simulink model "SpeedGoat_GridModel"  (R2024a)
settings: Solver=FixedStepDiscrete  StartTime=0.0  StopTime=inf  RelTol=1e-3
StopFcn:
  | Root = pwd; PathTestResult = fullfile(Root, 'TestCases', 'TestResults'); ModelParam = struct(); if exist('Sim', 'var'), ModelParam.Sim = Sim; end; if exist('Hil', 'var'), ModelParam.Hil = Hil; end; if exist('out', 'var'),     saveTestResults(out, 'Speedgoat', 'Meas', PathTestResult, 1, ModelParam); else,     disp('Warning: Simulation output "out" not found in workspace after stop.'); end
values from neighbouring files (symbols this model uses):
  Hil = 100.0    [ModelDD.sldd]
  Sim : value not decoded    [ModelDD.sldd]
undefined symbols (not defined in the file or in its folder): DiscIntNeverNeededParam, Ended, IO324, IO3xx, pull, Single, up
libraries: speedgoatlib_fpga_pwm x5, speedgoatlib_fpga_analog_io x5, speedgoatlib_fpga_dio x3, simulink x3, speedgoatlib_fpga_inta x1, speedgoatlib_interrupt x1, speedgoatlib_fpga_quadrature x1, speedgoatlib_fpga_spi x1, dspswit3 x1, slrealtimeloglib x1, slrealtimetgmanagement x1, simulink_extras x1
settings Model: SimulationMode=external  ExtModeEnableFloating=off  Creator=simon.beck  LastModifiedBy=The Professionals
settings SolverCC: ConcurrentTasks=on  PositivePriorityOrder=on
settings DataIOCC: LimitDataPoints=on  SaveFormat=StructureWithTime  SaveOutput=off  DSMLogging=off  StreamToWks=off  SaveTime=off
settings OptimizationCC: BlockReduction=off  OptimizeBlockIOStorage=off  BufferReuse=off  ReuseModelBlockBuffer=off
settings DebuggingCC: UnderspecifiedInitializationDetection=Classic  MergeDetectMultiDrivingBlocksExec=none  TasksWithSamePriorityMsg=none  ParameterDowncastMsg=warning  ParameterOverflowMsg=warning  FcnCallInpInsideContextMsg=warning  FrameProcessingCompatibilityMsg=warning  NonCurrentReleaseOperatingPointMsg=warning  SFUnexpectedBacktrackingDiag=warning  SFOutputUsedAsStateInMooreChartDiag=warning
settings HardwareCC: ProdBitPerLong=64  ProdLongLongMode=on  ProdHWDeviceType=Intel->x86-64 (Linux 64)
settings ModelReferenceCC: EnableRefExpFcnMdlSchedulingChecks=on  PropagateSignalLabelsOutOfModel=off
settings RTWCC: Description=Speedgoat Real-Time Target Machine  SystemTargetFile=speedgoat.tlc  TemplateMakefile=slrealtime_default_tmf  PostCodeGenCommand=sg.model.build.makeCfg(bdroot, buildInfo);  Toolchain=Simulink Real-Time Toolchain  BuildConfiguration=Faster Runs  CodeExecutionProfiling=on  TargetLang=C++  GPUComputeCapability=3.5
settings SimulinkRealTimeTargetCC: InstructionSetFMA=off  LogToMDFFile=off

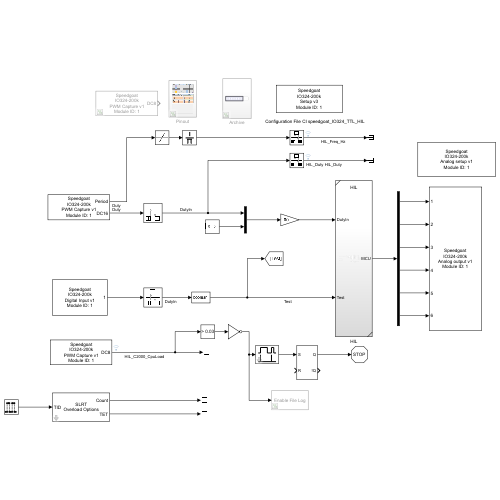
[thumbnail: Simulink's stored preview of the top-level diagram]
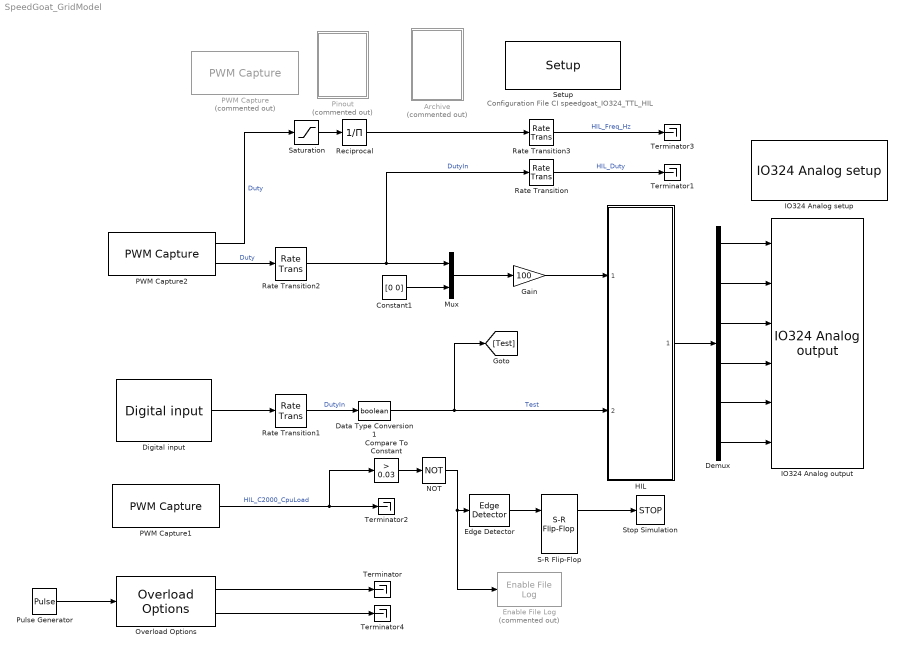
== system SpeedGoat_GridModel ==
  note: Configuration File CI speedgoat_IO324_TTL_HIL
  Archive : Subsystem  Commented=on
  Compare To Constant : simulink/Logic and Bit Operations/Compare To Constant  relop=>  const=0.03  OutDataTypeStr=boolean
  Constant1 : Constant  Value=[0 0]
  Data Type Conversion1 : DataTypeConversion  OutDataTypeStr=boolean  SaturateOnIntegerOverflow=off  RndMeth=Floor
  Demux : Demux  Outputs=6
  Digital input : speedgoatlib_fpga_dio/Digital input  id=1  chan=[1]  ts=1/Hil.PWM_Freq  vectorizeOutput=off
      settings: SourceProductName=Digital
  Edge Detector : dspswit3/Edge Detector  InputProcessing=Columns as channels (frame based)
  Enable File Log : slrealtimeloglib/Enable File Log  Commented=on
  Gain : Gain  Gain=100
  HIL : Subsystem  VariantControl="Sim.PlantOrMeas == \"HIL1\""  ReferencedSubsystem=HIL
  IO324 Analog output : speedgoatlib_fpga_analog_io/IO324/IO324 Analog output  id=1  parSampleTime=Sim.ContSampleTime  parPciSlot=-1  parAoChannels=[1 2 3 4 5 6]  parAoVoltageRange=[2 2 2 2 2 2]  parDacOverRange=[0 0 0 0 0 0 0 0]  parAoInitValues=[0 0 0 0 0 0]  parAoReset=[1 1 1 1 1 1]  parDacSyncOut=1  parAoEnableFrame=0  parDacActiveDmaDevices=[1 1 1 1]  parDacDmaLatency=2  parAoFrameSize=100
      settings: SourceProductName=Analog IO
  IO324 Analog setup : speedgoatlib_fpga_analog_io/IO324/IO324 Analog setup  id=1  parEnableCodeModule1=off  parEnableCodeModule2=off  parEnableCodeModule3=off  parEnableCodeModule4=off  parEnableCodeModule5=off  parEnableCodeModule6=off  parEnableCodeModule7=off  parEnableCodeModule8=off  parAdcEnableIndividualTrigger=off  parAdcTriggerMode1=Model Step  parAdcSampleRate1=100e3  parAdcDioTriggerChannel1=1  parAdcInternalTrigger1=<empty>  parAdcOversampling1=None  parAdcTriggerMode2=Model Step  parAdcSampleRate2=100e3  parAdcDioTriggerChannel2=1  parAdcInternalTrigger2=<empty>  parAdcOversampling2=None  parAdcTriggerMode3=Model Step  parAdcSampleRate3=100e3  parAdcDioTriggerChannel3=1  parAdcInternalTrigger3=<empty>  parAdcOversampling3=None  parAdcTriggerMode4=Model Step  parAdcSampleRate4=100e3  parAdcDioTriggerChannel4=1  parAdcInternalTrigger4=<empty>  parAdcOversampling4=None  parAdcReadPrevValueIndividualTrigger=on  parAdcEnableFrame=off  parAdcTriggerMode=Model Step  parAdcReadPrevValue=off  parAdcSampleRate=100e3  parAdcDioTriggerChannel=1  parAdcInternalTrigger=<empty>  parAdcOversampling=None  parAdcTriggerResolution=1e-08  parAdcSampleRateFrame=1000  parAdcFrameSize=100  parAdcSampleTime=-1  parDacTriggerMode=Model Step  parDacInternalTrigger=<empty>  parDacDioTriggerChannel=0  parDacEnableFrame=off  parDacFifoThreshold=100  parDacTriggerResolution=1e-08  parDacSampleRate=1000  parDacFrameSize=100  parDacSampleTime=-1  parAdcCoupling1=Differential  parAdcChannel1=on  parAdcChannel2=off  parAdcChannel3=on  parAdcChannel4=off  parAdcChannel5=off  parAdcChannel6=off  parAdcChannel7=off  parAdcChannel8=off  parAdcRangeAll1=+-10.24 V  parVoltageRangePerChannelEn1=off  parAdcRange1=+-10.24 V  parAdcRange5=+-10.24 V  parAdcRange2=+-10.24 V  parAdcRange6=+-10.24 V  parAdcRange3=+-10.24 V  parAdcRange7=+-10.24 V  parAdcRange4=+-10.24 V  parAdcRange8=+-10.24 V  parAdcCoupling2=Differential  parAdcChannel9=on  parAdcChannel10=off  parAdcChannel11=on  parAdcChannel12=off  parAdcChannel13=off  parAdcChannel14=off  parAdcChannel15=off  parAdcChannel16=off  parAdcRangeAll2=+-10.24 V  parVoltageRangePerChannelEn2=off  parAdcRange9=+-10.24 V  parAdcRange13=+-10.24 V  parAdcRange10=+-10.24 V  parAdcRange14=+-10.24 V  parAdcRange11=+-10.24 V  parAdcRange15=+-10.24 V  parAdcRange12=+-10.24 V  parAdcRange16=+-10.24 V  parAdcCoupling3=Single-Ended  parAdcChannel17=on  parAdcChannel18=on  parAdcChannel19=off  parAdcChannel20=off  parAdcChannel21=off  parAdcChannel22=off  parAdcChannel23=off  parAdcChannel24=off  parAdcRangeAll3=+-10.24 V  parVoltageRangePerChannelEn3=off  parAdcRange17=+-10.24 V  parAdcRange21=+-10.24 V  parAdcRange18=+-10.24 V  parAdcRange22=+-10.24 V  parAdcRange19=+-10.24 V  parAdcRange23=+-10.24 V  parAdcRange20=+-10.24 V  parAdcRange24=+-10.24 V  parAdcCoupling4=Single-Ended  parAdcChannel25=on  parAdcChannel26=on  parAdcChannel27=off  parAdcChannel28=off  parAdcChannel29=off  parAdcChannel30=off  parAdcChannel31=off  parAdcChannel32=off  parAdcRangeAll4=+-10.24 V  parVoltageRangePerChannelEn4=off  parAdcRange25=+-10.24 V  parAdcRange29=+-10.24 V  parAdcRange26=+-10.24 V  parAdcRange30=+-10.24 V  parAdcRange27=+-10.24 V  parAdcRange31=+-10.24 V  parAdcRange28=+-10.24 V  parAdcRange32=+-10.24 V  parAdcAutoCorrection=on  parDacChannel1=on  parDacChannel2=on  parDacChannel3=on  parDacChannel4=on  parDacChannel5=on  parDacChannel6=on  parDacChannel7=off  parDacChannel8=off  parDacRange1=+-5 V  parDacInitValue1=0  parDacReset1=on  parDacRange2=+-5 V  parDacInitValue2=0  parDacReset2=on  parDacRange3=+-5 V  parDacInitValue3=0  parDacReset3=on  parDacRange4=+-5 V  parDacInitValue4=0  parDacReset4=on  parDacRange5=+-5 V  parDacInitValue5=0  parDacReset5=on  parDacRange6=+-5 V  parDacInitValue6=0  parDacReset6=on  parDacRange7=+-5 V  parDacInitValue7=0  parDacReset7=on  parDacRange8=+-5 V  parDacInitValue8=0  parDacReset8=on  parDacAutoCorrection=on
      settings: SourceProductName=Analog IO
  Mux : Mux  Inputs=2
  NOT : Logic  Operator=NOT  IconShape=distinctive  AllPortsSameDT=off  OutDataTypeStr=boolean
  Overload Options : slrealtimetgmanagement/Overload Options  startupDur=1  startupDurSrc=Tunable Parameter  maxOverload=1e6  maxOverloadSrc=Tunable Parameter  TETFlag=on
  PWM Capture : speedgoatlib_fpga_pwm/PWM Capture  Commented=on  id=1  chan=[2 3 4 5]  ts=Sim.ContSampleTime  enableDma=on  captureMode=Use dedicated trigger input  bit_width_cap=24  captureTimeout_si=0  captureTimeout_eff=[0]  debounce_si=0.5e-6  debounce_eff=[500e-9]  showHighDuration=off  showLowDuration=off  showPeriod=off  showDC16=off  showDC8=on  showTOn=off  showTOff=off  showValidData=off
      settings: SourceProductName=PWM
  PWM Capture1 : speedgoatlib_fpga_pwm/PWM Capture  id=1  chan=[1]  ts=1/Hil.PWM_Freq  enableDma=on  captureMode=High transitions triggered  bit_width_cap=24  captureTimeout_si=0  captureTimeout_eff=[0]  debounce_si=0.5e-6  debounce_eff=[500e-9]  showHighDuration=off  showLowDuration=off  showPeriod=off  showDC16=off  showDC8=on  showTOn=off  showTOff=off  showValidData=off
      settings: SourceProductName=PWM
  PWM Capture2 : speedgoatlib_fpga_pwm/PWM Capture  id=1  chan=[2 3 4 5]  ts=1/Hil.PWM_Freq  enableDma=on  captureMode=Software triggered  bit_width_cap=24  captureTimeout_si=0  captureTimeout_eff=[0]  debounce_si=0.5e-6  debounce_eff=[500e-9]  showHighDuration=off  showLowDuration=off  showPeriod=on  showDC16=on  showDC8=off  showTOn=off  showTOff=off  showValidData=off
      settings: SourceProductName=PWM
  Pinout : Subsystem  Commented=on
  Pulse Generator : DiscretePulseGenerator  Period=10  PulseWidth=5  SampleTime=Sim.ContSampleTime
  Rate Transition : RateTransition  OutPortSampleTime=Hil.MeasSlowSmplTime
  Rate Transition1 : RateTransition
  Rate Transition2 : RateTransition
  Rate Transition3 : RateTransition  OutPortSampleTime=Hil.MeasSlowSmplTime
  Reciprocal : Product  Inputs=/
  S-R Flip-Flop : simulink_extras/Flip Flops/S-R Flip-Flop  initial_condition=0
  Saturation : Saturate  UpperLimit=inf  LowerLimit=eps
  Setup : speedgoatlib_fpga/Setup/Setup  Parameter124={}  board=IO324-200k  id=1  pciSlot=-1  device_id=1  bitstreamFilePath=C:\ProgramData\Speedgoat\bitstreams\io_configuration_package\R2024a\io324  bitstreamFile=speedgoat_IO324_21_TTL_HIL.mat  rearEnb_1=off  rearIO_1=IO3xx-21  rearEnb_2=off  rearIO_2=None  ProgSpiFlash=off  ProgBPIFlash=off  useFpgaDmaController=off  PullRPort15=pull-down  PullRPort31=pull-down  PullRPort47=pull-up 3.3V  PullRPort63=pull-up 3.3V  diffLineTermination_1=on  diffLineTermination_2=on  diffLineTermination_3=on  diffLineTermination_4=on  diffLineTermination_5=on  diffLineTermination_6=on  diffLineTermination_7=on  diffLineTermination_8=on  diffLineTermination_9=on  diffLineTermination_10=on  diffLineTermination_11=on  diffLineTermination_12=on  diffLineTermination_13=on  diffLineTermination_14=on  diffLineTermination_15=on  diffLineTermination_16=on  diffLineTermination_17=on  diffLineTermination_18=on  diffLineTermination_19=on  diffLineTermination_20=on  diffLineTermination_21=on  diffLineTermination_22=on  diffLineTermination_23=on  diffLineTermination_24=on  diffLineTermination_25=on  diffLineTermination_26=on  diffLineTermination_27=on  diffLineTermination_28=on  diffLineTermination_29=on  diffLineTermination_30=on  diffLineTermination_31=on  diffLineTermination_32=on  Vi_Pull_36x_1=Floating  Vo_36x_1=3.3V  Vi_Pull_36x_2=Floating  Vo_36x_2=3.3V  Vi_Pull_36x_3=Floating  Vo_36x_3=3.3V  Vi_Pull_36x_4=Floating  Vo_36x_4=3.3V  Vi_Pull_36x_5=Floating  Vo_36x_5=3.3V  Vi_Pull_36x_6=Floating  Vo_36x_6=3.3V  Vi_Pull_36x_7=Floating  Vo_36x_7=3.3V  Vi_Pull_36x_8=Floating  Vo_36x_8=3.3V  Vi_Pull_36x_9_16=Floating  Vo_36x_9_16=3.3V  Vi_Pull_36x_17_24=Floating  Vo_36x_17_24=3.3V  Vi_Pull_36x_25_32=Floating  Vo_36x_25_32=3.3V  Vi_Pull_36x_33_40=Floating  Vo_36x_33_40=3.3V  Vi_Pull_36x_41_48=Floating  Vo_36x_41_48=3.3V  Vi_Pull_36x_49_56=Floating  Vo_36x_49_56=3.3V  Vi_Pull_36x_57_64=Floating  Vo_36x_57_64=3.3V  PullRPort0_1=pull-up  VioPort0_1=5.0V  PullRPort1_1=pull-up  VioPort1_1=3.3V  PullRPort2_1=pull-up  VioPort2_1=3.3V  PullRPort3_1=pull-up  VioPort3_1=3.3V  PullRPort4_1=pull-up  VioPort4_1=3.3V  PullRPort5_1=pull-up  VioPort5_1=3.3V  PullRPort6_1=pull-up  VioPort6_1=3.3V  diffLineTermination_rear1_1=on  diffLineTermination_rear1_2=on  diffLineTermination_rear1_3=on  diffLineTermination_rear1_4=on  diffLineTermination_rear1_5=on  diffLineTermination_rear1_6=on  diffLineTermination_rear1_7=on  diffLineTermination_rear1_8=on  PullRPort0_2=pull-up  VioPort0_2=3.3V  PullRPort1_2=pull-up  VioPort1_2=3.3V  PullRPort2_2=pull-up  VioPort2_2=3.3V  PullRPort3_2=pull-up  VioPort3_2=3.3V  PullRPort4_2=pull-up  VioPort4_2=3.3V  PullRPort5_2=pull-up  VioPort5_2=3.3V  PullRPort6_2=pull-up  VioPort6_2=3.3V  diffLineTermination_rear2_1=on  diffLineTermination_rear2_2=on  diffLineTermination_rear2_3=on  diffLineTermination_rear2_4=on  diffLineTermination_rear2_5=on  diffLineTermination_rear2_6=on  diffLineTermination_rear2_7=on  diffLineTermination_rear2_8=on
      settings: SourceProductName=IO3xx
  Stop Simulation : Stop
  Terminator{,1..4} (5 alike) : Terminator
  wires:
  PWM Capture2/2 -> Rate Transition2/1  "Duty"
  Rate Transition2/1 -> Mux/1, Rate Transition/1  "DutyIn"
  Overload Options/1 -> Terminator/1
  Rate Transition/1 -> Terminator1/1  "HIL_Duty"
  Digital input/1 -> Rate Transition1/1
  Data Type Conversion1/1 -> HIL/2, [Test]  "Test"
  Demux/2 -> IO324 Analog output/2
  Demux/4 -> IO324 Analog output/4
  PWM Capture1/1 -> Compare To Constant/1, Terminator2/1  "HIL_C2000_CpuLoad"
  Demux/1 -> IO324 Analog output/1
  Demux/3 -> IO324 Analog output/3
  Demux/5 -> IO324 Analog output/5
  Demux/6 -> IO324 Analog output/6
  Pulse Generator/1 -> Overload Options/1
  HIL/1 -> Demux/1
  Constant1/1 -> Mux/2
  Mux/1 -> Gain/1
  Gain/1 -> HIL/1
  Rate Transition1/1 -> Data Type Conversion1/1  "DutyIn"
  Rate Transition3/1 -> Terminator3/1  "HIL_Freq_Hz"
  PWM Capture2/1 -> Saturation/1  "Duty"
  Reciprocal/1 -> Rate Transition3/1
  Overload Options/2 -> Terminator4/1
  Saturation/1 -> Reciprocal/1
  Edge Detector/1 -> S-R Flip-Flop/1
  S-R Flip-Flop/1 -> Stop Simulation/1
  NOT/1 -> Enable File Log/1, Edge Detector/1
  Compare To Constant/1 -> NOT/1

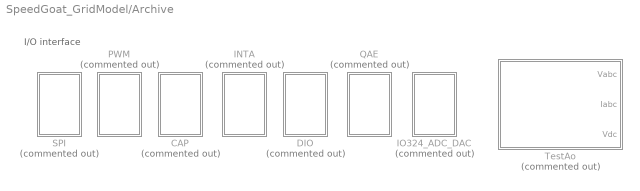
== system SpeedGoat_GridModel/Archive ==
  note: I/O interface
  CAP : Subsystem  Commented=on
  DIO : Subsystem  Commented=on
  INTA : Subsystem  Commented=on
  IO324_ADC_DAC : Subsystem  Commented=on
  PWM : Subsystem  Commented=on
  QAE : Subsystem  Commented=on
  SPI : Subsystem  Priority=1  Commented=on
  TestAo : Subsystem  Commented=on

== system SpeedGoat_GridModel/Pinout ==

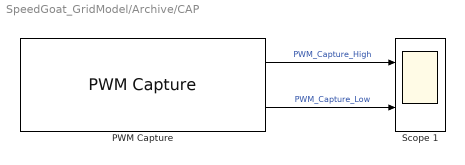
== system SpeedGoat_GridModel/Archive/CAP ==
  PWM Capture : speedgoatlib_fpga_pwm/PWM Capture  id=1  chan=[4 5]  ts=Sim.ContSampleTime  enableDma=on  captureMode=Use dedicated trigger input  bit_width_cap=24  captureTimeout_si=0  captureTimeout_eff=[0]  debounce_si=0.5e-6  debounce_eff=[500e-9]  showHighDuration=on  showLowDuration=on  showPeriod=off  showDC16=off  showDC8=off  showTOn=off  showTOff=off  showValidData=off
      settings: SourceProductName=PWM
  "Scope 1 " : Scope  NumInputPorts=2
  wires:
  PWM Capture/1 -> "Scope 1 "/1  "PWM_Capture_High"
  PWM Capture/2 -> "Scope 1 "/2  "PWM_Capture_Low"

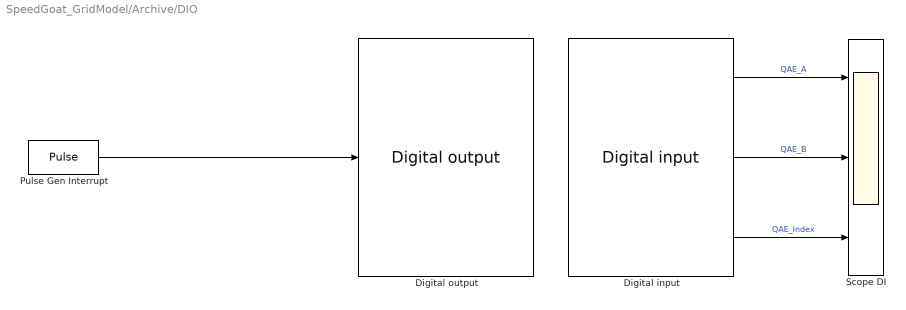
== system SpeedGoat_GridModel/Archive/DIO ==
  Digital input : speedgoatlib_fpga_dio/Digital input  id=1  chan=[30:32]  ts=Sim.ContSampleTime  vectorizeOutput=off
      settings: SourceProductName=Digital
  Digital output : speedgoatlib_fpga_dio/Digital output  id=1  chan=[9]  init=[0]  reset=[0]  ts=Sim.ContSampleTime  vectorizeInput=off
      settings: SourceProductName=Digital
  Pulse Gen Interrupt : DiscretePulseGenerator  PhaseDelay=[0]  SampleTime=Sim.ContSampleTime  VectorParams1D=off
  Scope DI : Scope  NumInputPorts=3
  wires:
  Digital input/1 -> Scope DI/1  "QAE_A"
  Pulse Gen Interrupt/1 -> Digital output/1
  Digital input/2 -> Scope DI/2  "QAE_B"
  Digital input/3 -> Scope DI/3  "QAE_Index"

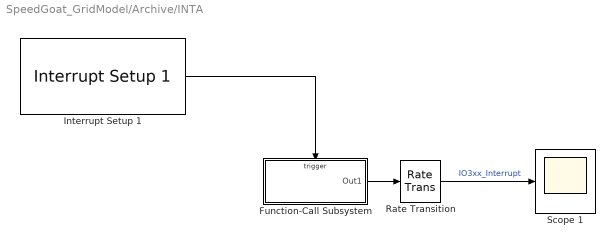
== system SpeedGoat_GridModel/Archive/INTA ==
  Function-Call Subsystem : Subsystem  TreatAsAtomicUnit=on
  Interrupt Setup 1 : speedgoatlib_interrupt/Interrupt Setup 1  parModuleTrigger=off  parPollingMode=off  parPriorityConf=High  parPriority=241  confStartFcn=IO324_200k_start_public  confStopFcn=IO324_200k_stop_public  confIsrFcn=IO324_200k_isr_public  confMapFcn=IO324_200k_map_public  confHookFile=io324_200k_int_hooks.c  confIrqNr=-1  confIsPolling=off  confModID=16776961  confSelectedInt=Speedgoat IO324-200k interrupt  confSelectedId=1  confSelectedChannel=[]
  Rate Transition : RateTransition  Integrity=off
  "Scope 1 " : Scope
  wires:
  Rate Transition/1 -> "Scope 1 "/1  "IO3xx_Interrupt"
  Function-Call Subsystem/1(Out1) -> Rate Transition/1
  Interrupt Setup 1/1 -> Function-Call Subsystem/Trigger

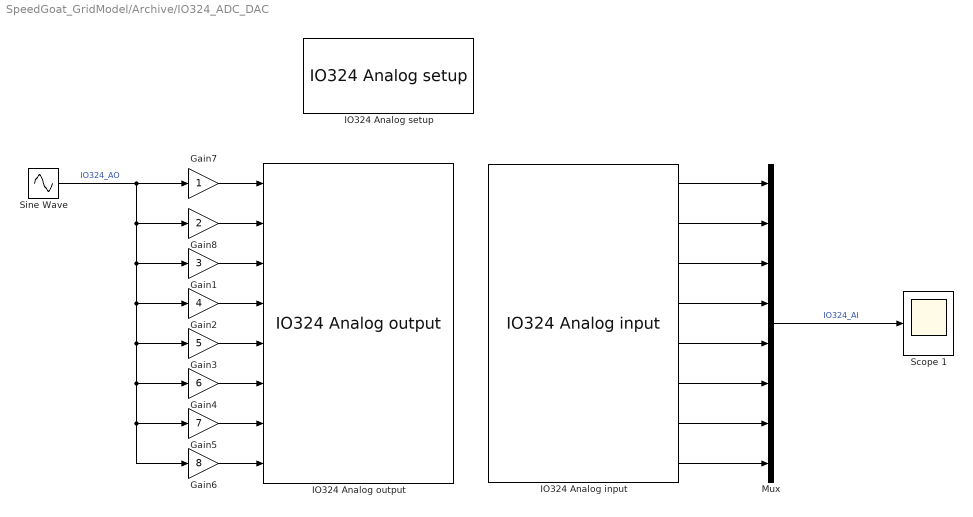
== system SpeedGoat_GridModel/Archive/IO324_ADC_DAC ==
  Gain1 : Gain  Gain=3
  Gain2 : Gain  Gain=4
  Gain3 : Gain  Gain=5
  Gain4 : Gain  Gain=6
  Gain5 : Gain  Gain=7
  Gain6 : Gain  Gain=8
  Gain7 : Gain
  Gain8 : Gain  Gain=2
  IO324 Analog input : speedgoatlib_fpga_analog_io/IO324/IO324 Analog input  id=1  parSampleTime=Sim.ContSampleTime  parPciSlot=-1  parAiChannels=[1 3 9 11 17 18 25 26]  parAiTriggerMode=[1 1 1 1]  parAiReadPrevValue=0  parAiEnableFrame=0  parAiVoltageRange=[2 2 2 2 2 2 2 2]  parAdcCoupling=[1 1 1 1]  parAdcContSampling=0  parAdcDmaEnable=0  parAdcActiveDmaDevices=[1 1 1 1]  parAiFrameSize=100
      settings: SourceProductName=Analog IO
  IO324 Analog output : speedgoatlib_fpga_analog_io/IO324/IO324 Analog output  id=1  parSampleTime=Sim.ContSampleTime  parPciSlot=-1  parAoChannels=[1 2 3 4 5 6 7 8]  parAoVoltageRange=[1 1 1 1 1 1 1 1]  parDacOverRange=[0 0 0 0 0 0 0 0]  parAoInitValues=[0 0 0 0 0 0 0 0]  parAoReset=[1 1 1 1 1 1 1 1]  parDacSyncOut=1  parAoEnableFrame=0  parDacActiveDmaDevices=[1 1 1 1]  parDacDmaLatency=2  parAoFrameSize=100
      settings: SourceProductName=Analog IO
  IO324 Analog setup : speedgoatlib_fpga_analog_io/IO324/IO324 Analog setup  id=1  parEnableCodeModule1=off  parEnableCodeModule2=off  parEnableCodeModule3=off  parEnableCodeModule4=off  parEnableCodeModule5=off  parEnableCodeModule6=off  parEnableCodeModule7=off  parEnableCodeModule8=off  parAdcEnableIndividualTrigger=off  parAdcTriggerMode1=Model Step  parAdcSampleRate1=100e3  parAdcDioTriggerChannel1=1  parAdcInternalTrigger1=<empty>  parAdcOversampling1=None  parAdcTriggerMode2=Model Step  parAdcSampleRate2=100e3  parAdcDioTriggerChannel2=1  parAdcInternalTrigger2=<empty>  parAdcOversampling2=None  parAdcTriggerMode3=Model Step  parAdcSampleRate3=100e3  parAdcDioTriggerChannel3=1  parAdcInternalTrigger3=<empty>  parAdcOversampling3=None  parAdcTriggerMode4=Model Step  parAdcSampleRate4=100e3  parAdcDioTriggerChannel4=1  parAdcInternalTrigger4=<empty>  parAdcOversampling4=None  parAdcReadPrevValueIndividualTrigger=on  parAdcEnableFrame=off  parAdcTriggerMode=Model Step  parAdcReadPrevValue=off  parAdcSampleRate=100e3  parAdcDioTriggerChannel=1  parAdcInternalTrigger=<empty>  parAdcOversampling=None  parAdcTriggerResolution=1e-08  parAdcSampleRateFrame=1000  parAdcFrameSize=100  parAdcSampleTime=-1  parDacTriggerMode=Model Step  parDacInternalTrigger=<empty>  parDacDioTriggerChannel=0  parDacEnableFrame=off  parDacFifoThreshold=100  parDacTriggerResolution=1e-08  parDacSampleRate=1000  parDacFrameSize=100  parDacSampleTime=-1  parAdcCoupling1=Differential  parAdcChannel1=on  parAdcChannel2=off  parAdcChannel3=on  parAdcChannel4=off  parAdcChannel5=off  parAdcChannel6=off  parAdcChannel7=off  parAdcChannel8=off  parAdcRangeAll1=+-10.24 V  parVoltageRangePerChannelEn1=off  parAdcRange1=+-10.24 V  parAdcRange5=+-10.24 V  parAdcRange2=+-10.24 V  parAdcRange6=+-10.24 V  parAdcRange3=+-10.24 V  parAdcRange7=+-10.24 V  parAdcRange4=+-10.24 V  parAdcRange8=+-10.24 V  parAdcCoupling2=Differential  parAdcChannel9=on  parAdcChannel10=off  parAdcChannel11=on  parAdcChannel12=off  parAdcChannel13=off  parAdcChannel14=off  parAdcChannel15=off  parAdcChannel16=off  parAdcRangeAll2=+-10.24 V  parVoltageRangePerChannelEn2=off  parAdcRange9=+-10.24 V  parAdcRange13=+-10.24 V  parAdcRange10=+-10.24 V  parAdcRange14=+-10.24 V  parAdcRange11=+-10.24 V  parAdcRange15=+-10.24 V  parAdcRange12=+-10.24 V  parAdcRange16=+-10.24 V  parAdcCoupling3=Single-Ended  parAdcChannel17=on  parAdcChannel18=on  parAdcChannel19=off  parAdcChannel20=off  parAdcChannel21=off  parAdcChannel22=off  parAdcChannel23=off  parAdcChannel24=off  parAdcRangeAll3=+-10.24 V  parVoltageRangePerChannelEn3=off  parAdcRange17=+-10.24 V  parAdcRange21=+-10.24 V  parAdcRange18=+-10.24 V  parAdcRange22=+-10.24 V  parAdcRange19=+-10.24 V  parAdcRange23=+-10.24 V  parAdcRange20=+-10.24 V  parAdcRange24=+-10.24 V  parAdcCoupling4=Single-Ended  parAdcChannel25=on  parAdcChannel26=on  parAdcChannel27=off  parAdcChannel28=off  parAdcChannel29=off  parAdcChannel30=off  parAdcChannel31=off  parAdcChannel32=off  parAdcRangeAll4=+-10.24 V  parVoltageRangePerChannelEn4=off  parAdcRange25=+-10.24 V  parAdcRange29=+-10.24 V  parAdcRange26=+-10.24 V  parAdcRange30=+-10.24 V  parAdcRange27=+-10.24 V  parAdcRange31=+-10.24 V  parAdcRange28=+-10.24 V  parAdcRange32=+-10.24 V  parAdcAutoCorrection=on  parDacChannel1=on  parDacChannel2=on  parDacChannel3=on  parDacChannel4=on  parDacChannel5=on  parDacChannel6=on  parDacChannel7=on  parDacChannel8=on  parDacRange1=+-10 V  parDacInitValue1=0  parDacReset1=on  parDacRange2=+-10 V  parDacInitValue2=0  parDacReset2=on  parDacRange3=+-10 V  parDacInitValue3=0  parDacReset3=on  parDacRange4=+-10 V  parDacInitValue4=0  parDacReset4=on  parDacRange5=+-10 V  parDacInitValue5=0  parDacReset5=on  parDacRange6=+-10 V  parDacInitValue6=0  parDacReset6=on  parDacRange7=+-10 V  parDacInitValue7=0  parDacReset7=on  parDacRange8=+-10 V  parDacInitValue8=0  parDacReset8=on  parDacAutoCorrection=on
      settings: SourceProductName=Analog IO
  Mux : Mux  Inputs=8
  "Scope 1 " : Scope
  Sine Wave : Sin  SineType=Sample based  Frequency=2*pi*(1/Sim.ContSampleTime)/50  Samples=1000  SampleTime=Sim.ContSampleTime
  wires:
  IO324 Analog input/1 -> Mux/1
  Mux/1 -> "Scope 1 "/1  "IO324_AI"
  IO324 Analog input/2 -> Mux/2
  IO324 Analog input/3 -> Mux/3
  IO324 Analog input/4 -> Mux/4
  IO324 Analog input/5 -> Mux/5
  IO324 Analog input/6 -> Mux/6
  IO324 Analog input/7 -> Mux/7
  IO324 Analog input/8 -> Mux/8
  Sine Wave/1 -> Gain6/1, Gain5/1, Gain4/1, Gain3/1, Gain2/1, Gain1/1, Gain8/1, Gain7/1  "IO324_AO"
  Gain1/1 -> IO324 Analog output/3
  Gain2/1 -> IO324 Analog output/4
  Gain3/1 -> IO324 Analog output/5
  Gain4/1 -> IO324 Analog output/6
  Gain5/1 -> IO324 Analog output/7
  Gain6/1 -> IO324 Analog output/8
  Gain7/1 -> IO324 Analog output/1
  Gain8/1 -> IO324 Analog output/2

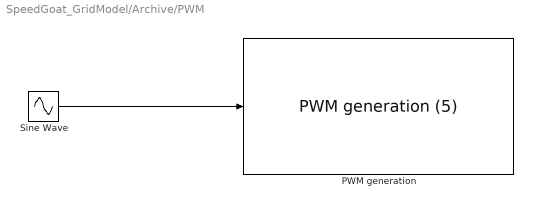
== system SpeedGoat_GridModel/Archive/PWM ==
  PWM generation : speedgoatlib_fpga_pwm/PWM generation (5)  id=1  chan=[1]  board=IO324-200k  ts=Sim.ContSampleTime  enableDma=off  pciSlot=[-1,-1]  delay=0  symmetric=Symmetric - PWM generation is centered around half the period  b_is_complement_of_a=The complement of PWM A output  deadband=[0.0]  period=[1/1000]  frequency=1000  ticks=99999  a_on=0  a_off=0.5e-3  pwm_a_dc=[0.0]  b_on=0.25e-3  b_off=0.75e-3  pwm_b_dc=[0]  c_on=[0.0]  c_off=[0.0]  protection=Disabled: A and B can be high at the same moment  enable_latch_half_period=off  pwm_update=At period starts  bit_width_pwm_gen=24  trigger_duration=[1e-6]  trigger_period_start=off  trigger_half_of_the_period=on  trigger_a_on=off  trigger_a_off=off  trigger_b_on=off  trigger_b_off=off  show_a_input=on  show_b_input=on  show_c_input=off  show_period_input=off  show_force_stop_input=off  idle_a=Low when PWM generation is halted  idle_b=Low when PWM generation is halted  idle_c=Low when PWM generation is halted  cancels_pwm_generation=on  invert_a=off  invert_b=off  invert_c=off
      settings: SourceProductName=PWM
  Sine Wave : Sin  SineType=Sample based  Amplitude=0.5  Bias=0.5  Samples=1000  SampleTime=Sim.ContSampleTime
  wires:
  Sine Wave/1 -> PWM generation/1

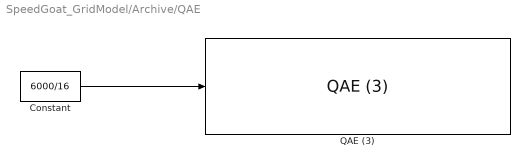
== system SpeedGoat_GridModel/Archive/QAE ==
  Constant : Constant  Value=6000/16  OutDataTypeStr=Inherit: Inherit via back propagation
  QAE (3) : speedgoatlib_fpga_quadrature/QAE (3)  id=1  chan=[2]  sampleTime=Sim.ContSampleTime  enableDma=on  numOfSlots=[16]  sigAswitchOn=[180]  sigBswitchOff=[90]  sigBswitchOn=[270]  initPos=0  sigAdismissEn=off  sigAdismissSingle=on  sigAdismissHigh=on  sigBdismissEn=off  sigBdismissSingle=on  sigBdismissHigh=on  showOutputPosition=off  showOutputSlotAngle=off
      settings: SourceProductName=Quadrature
  wires:
  Constant/1 -> QAE (3)/1

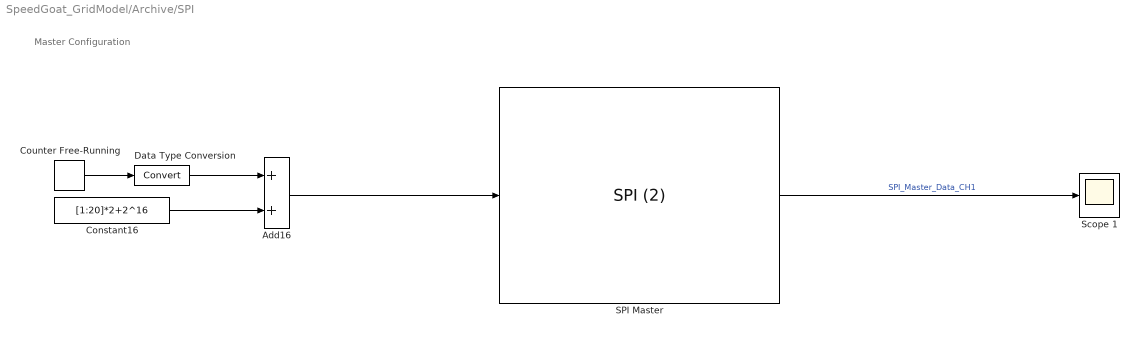
== system SpeedGoat_GridModel/Archive/SPI ==
  note: Master Configuration
  Add16 : Sum
  Constant16 : Constant  Value=[1:20]*2+2^16  OutDataTypeStr=Inherit: Inherit via back propagation
  Counter Free-Running : simulink/Sources/Counter Free-Running  NumBits=16  tsamp=-1
  Data Type Conversion : DataTypeConversion  SaturateOnIntegerOverflow=off  RndMeth=Floor
  SPI Master : speedgoatlib_fpga_spi/SPI (2)  Priority=1  id=1  chan=[1]  samp_time=Sim.ContSampleTime*10  role=Master  sync_mode=on  multislave_mode=off  write_only=off  read_only=off  enableDma=off  multislave_chan=[1:8]  cpol=[0]  cpha=[1]  frequency=[350e3]  frequency_eff=349.7e3  delay_start=[2e-6]  delay_start_eff=2e-6  delay_interword=[2e-6]  delay_interword_eff=2e-6  delay_stop=[2e-6]  delay_stop_eff=2e-6  delay_compensation=[100e-9]  delay_compensation_eff=100e-9  words_per_frame=[20]  dynamic_words_per_frame=off  bits_per_word=[20]  bit_shift_lsb_first=[1]  no_cs=off  clock_timeout=[1e-6]  clock_timeout_eff=1E-06
      settings: SourceProductName=SPI
  "Scope 1 " : Scope
  wires:
  Add16/1 -> SPI Master/1
  SPI Master/1 -> "Scope 1 "/1  "SPI_Master_Data_CH1"
  Constant16/1 -> Add16/2
  Counter Free-Running/1 -> Data Type Conversion/1
  Data Type Conversion/1 -> Add16/1

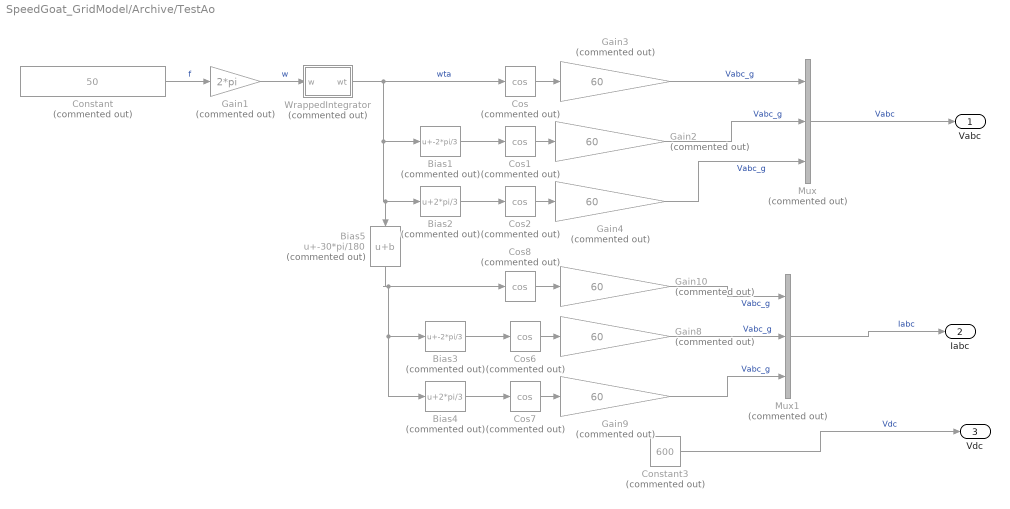
== system SpeedGoat_GridModel/Archive/TestAo ==
  Bias1 : Bias  Commented=on  Bias=-2*pi/3  SaturateOnIntegerOverflow=off
  Bias2 : Bias  Commented=on  Bias=2*pi/3  SaturateOnIntegerOverflow=off
  Bias3 : Bias  Commented=on  Bias=-2*pi/3  SaturateOnIntegerOverflow=off
  Bias4 : Bias  Commented=on  Bias=2*pi/3  SaturateOnIntegerOverflow=off
  Bias5 : Bias  Commented=on  Bias=-30*pi/180  SaturateOnIntegerOverflow=off
  Constant : Constant  Commented=on  Value=50
  Constant3 : Constant  Commented=on  Value=600
  Cos{,1..2,6..8} (6 alike) : Trigonometry  Commented=on  Operator=cos
  Gain1 : Gain  Commented=on  Gain=2*pi
  Gain{2..4,8..10} (6 alike) : Gain  Commented=on  Gain=60
  Mux : Mux  Commented=on  Inputs=3
  Mux1 : Mux  Commented=on  Inputs=3
  WrappedIntegrator : Subsystem  Commented=on
  Vabc : Outport
  Iabc : Outport  Port=2
  Vdc : Outport  Port=3
  wires:
  Bias1/1 -> Cos1/1
  Gain4/1 -> Mux/3  "Vabc_g"
  Constant3/1 -> Vdc/1  "Vdc"
  Bias3/1 -> Cos6/1
  Gain1/1 -> WrappedIntegrator/1(w)  "w"
  Cos1/1 -> Gain2/1
  Bias2/1 -> Cos2/1
  WrappedIntegrator/1(wt) -> Cos/1, Bias1/1, Bias2/1, Bias5/1  "wta"
  Gain2/1 -> Mux/2  "Vabc_g"
  Cos6/1 -> Gain8/1
  Cos2/1 -> Gain4/1
  Gain3/1 -> Mux/1  "Vabc_g"
  Bias4/1 -> Cos7/1
  Bias5/1 -> Cos8/1, Bias3/1, Bias4/1
  Mux/1 -> Vabc/1  "Vabc"
  Mux1/1 -> Iabc/1  "Iabc"
  Gain9/1 -> Mux1/3  "Vabc_g"
  Cos/1 -> Gain3/1
  Gain8/1 -> Mux1/2  "Vabc_g"
  Cos8/1 -> Gain10/1
  Cos7/1 -> Gain9/1
  Constant/1 -> Gain1/1  "f"
  Gain10/1 -> Mux1/1  "Vabc_g"

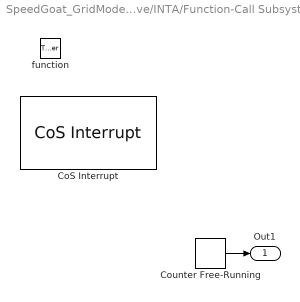
== system SpeedGoat_GridModel/Archive/INTA/Function-Call Subsystem ==
  function : TriggerPort  TriggerType=function-call  VariantControl=Variant
  CoS Interrupt : speedgoatlib_fpga_inta/CoS Interrupt  id=1  ts=-1  debounce=0  delay=0  polarity=1
      settings: SourceProductName=Interrupt
  Counter Free-Running : simulink/Sources/Counter Free-Running  NumBits=32  tsamp=-1
  Out1 : Outport  InitialOutput=[0]  VectorParamsAs1DForOutWhenUnconnected=off
  wires:
  Counter Free-Running/1 -> Out1/1

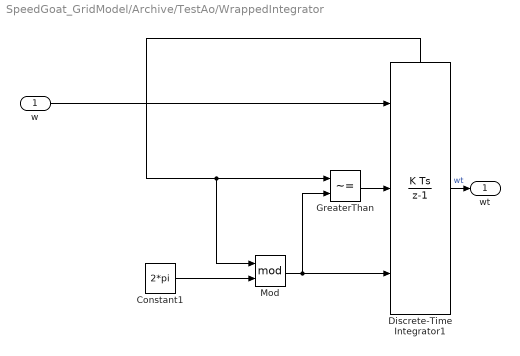
== system SpeedGoat_GridModel/Archive/TestAo/WrappedIntegrator ==
  w : Inport
  Constant1 : Constant  Value=2*pi
  Discrete-Time Integrator1 : DiscreteIntegrator  ExternalReset=rising  InitialConditionSource=external  SampleTime=-1  ShowStatePort=on  ICPrevOutput=DiscIntNeverNeededParam  ICPrevScaledInput=DiscIntNeverNeededParam
  GreaterThan : RelationalOperator  Operator=~=  OutDataTypeStr=boolean  RndMeth=Simplest  InputSameDT=off
  Mod : Math  Operator=mod
  wt : Outport
  wires:
  Constant1/1 -> Mod/2
  Mod/1 -> Discrete-Time Integrator1/3, GreaterThan/2
  Discrete-Time Integrator1/State -> GreaterThan/1, Mod/1
  w/1 -> Discrete-Time Integrator1/1
  Discrete-Time Integrator1/1 -> wt/1  "wt"
  GreaterThan/1 -> Discrete-Time Integrator1/2
